simulink model "Sim"  (R2016a)
settings: Solver=VariableStepAuto  StartTime=0.0  StopTime=1500  FixedStep=1  RelTol=1e-3
values from neighbouring files (symbols this model uses):
  A = 7.841E16    (= 7.841e+16)    [Parameters.m]
  cv = 1820000    [Parameters.m]
  detaX = 0.0013333    [Parameters.m]
  Ea = 1.4766E5    (= 147660)    [Parameters.m]
  H_dr = 4.92E8    (= 492000000)    [Parameters.m]
  H_pc = 1.992E8    (= 199200000)    [Parameters.m]
  ord = 0.75    [Parameters.m]
  q_dot = 3.981E4    (= 39810)    [Parameters.m]
  T_0 = 298.15    [Parameters.m]
  Tl = 334.15    [Parameters.m]
  Ts = 331.15    [Parameters.m]
(part 1 of 3)
settings Model: Creator=pc  LastModifiedBy=pc

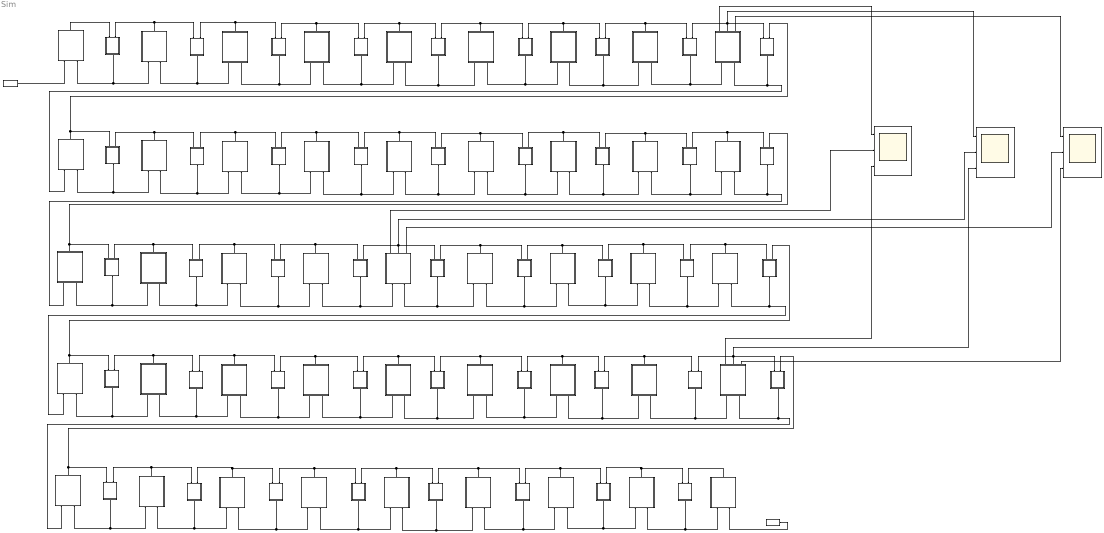
== system Sim ==
  Constant11 : Constant  Value=0
  Constant5 : Constant  Value=q_dot/detaX
  Element : Subsystem
  Element1 : Subsystem
  Element10 : Subsystem
  Element11 : Subsystem
  Element12 : Subsystem
  Element13 : Subsystem
  Element14 : Subsystem
  Element15 : Subsystem
  Element16 : Subsystem
  Element17 : Subsystem
  Element18 : Subsystem
  Element19 : Subsystem
  Element2 : Subsystem
  Element20 : Subsystem
  Element21 : Subsystem
  Element22 : Subsystem
  Element23 : Subsystem
  Element24 : Subsystem
  Element25 : Subsystem
  Element26 : Subsystem
  Element27 : Subsystem
  Element28 : Subsystem
  Element29 : Subsystem
  Element3 : Subsystem
  Element30 : Subsystem
  Element31 : Subsystem
  Element32 : Subsystem
  Element33 : Subsystem
  Element34 : Subsystem
  Element35 : Subsystem
  Element36 : Subsystem
  Element37 : Subsystem
  Element38 : Subsystem
  Element39 : Subsystem
  Element4 : Subsystem
  Element40 : Subsystem
  Element41 : Subsystem
  Element42 : Subsystem
  Element43 : Subsystem
  Element44 : Subsystem
  Element5 : Subsystem
  Element6 : Subsystem
  Element7 : Subsystem
  Element8 : Subsystem
  Element9 : Subsystem
  Heat treansfer : Subsystem
  Heat treansfer1 : Subsystem
  Heat treansfer10 : Subsystem
  Heat treansfer11 : Subsystem
  Heat treansfer12 : Subsystem
  Heat treansfer13 : Subsystem
  Heat treansfer14 : Subsystem
  Heat treansfer15 : Subsystem
  Heat treansfer16 : Subsystem
  Heat treansfer17 : Subsystem
  Heat treansfer18 : Subsystem
  Heat treansfer19 : Subsystem
  Heat treansfer2 : Subsystem
  Heat treansfer20 : Subsystem
  Heat treansfer21 : Subsystem
  Heat treansfer22 : Subsystem
  Heat treansfer23 : Subsystem
  Heat treansfer24 : Subsystem
  Heat treansfer25 : Subsystem
  Heat treansfer26 : Subsystem
  Heat treansfer27 : Subsystem
  Heat treansfer28 : Subsystem
  Heat treansfer29 : Subsystem
  Heat treansfer3 : Subsystem
  Heat treansfer30 : Subsystem
  Heat treansfer31 : Subsystem
  Heat treansfer32 : Subsystem
  Heat treansfer33 : Subsystem
  Heat treansfer34 : Subsystem
  Heat treansfer35 : Subsystem
  Heat treansfer36 : Subsystem
  Heat treansfer37 : Subsystem
  Heat treansfer38 : Subsystem
  Heat treansfer39 : Subsystem
  Heat treansfer4 : Subsystem
  Heat treansfer40 : Subsystem
  Heat treansfer41 : Subsystem
  Heat treansfer42 : Subsystem
  Heat treansfer44 : Subsystem
  Heat treansfer5 : Subsystem
  Heat treansfer6 : Subsystem
  Heat treansfer7 : Subsystem
  Heat treansfer8 : Subsystem
  Heat treansfer9 : Subsystem
  Scope : Scope  NumInputPorts=3
  Scope1 : Scope  NumInputPorts=3
  Scope2 : Scope  NumInputPorts=3
  wires:
  Constant5/1 -> Element/1(Q_in)  "Q_in"
  Element1/2(Temp) -> Heat treansfer1/1(Temp(+)), Heat treansfer/2(Temp(-))
  Heat treansfer/1(Q[W/m3]) -> Element1/1(Q_in), Element/2(Q_out)
  Heat treansfer1/1(Q[W/m3]) -> Element2/1(Q_in), Element1/2(Q_out)
  Heat treansfer2/1(Q[W/m3]) -> Element3/1(Q_in), Element2/2(Q_out)
  Heat treansfer3/1(Q[W/m3]) -> Element4/1(Q_in), Element3/2(Q_out)
  Heat treansfer4/1(Q[W/m3]) -> Element15/1(Q_in), Element4/2(Q_out)
  Element3/2(Temp) -> Heat treansfer2/2(Temp(-)), Heat treansfer3/1(Temp(+))
  Element2/2(Temp) -> Heat treansfer1/2(Temp(-)), Heat treansfer2/1(Temp(+))
  Heat treansfer14/1(Q[W/m3]) -> Element16/1(Q_in), Element15/2(Q_out)
  Heat treansfer15/1(Q[W/m3]) -> Element16/2(Q_out), Element17/1(Q_in)
  Element15/2(Temp) -> Heat treansfer14/1(Temp(+)), Heat treansfer4/2(Temp(-))
  Element16/2(Temp) -> Heat treansfer15/1(Temp(+)), Heat treansfer14/2(Temp(-))
  Element5/2(Temp) -> Heat treansfer17/2(Temp(-)), Heat treansfer5/1(Temp(+))
  Heat treansfer16/1(Q[W/m3]) -> Element18/1(Q_in), Element17/2(Q_out)
  Heat treansfer17/1(Q[W/m3]) -> Element5/1(Q_in), Element18/2(Q_out)
  Element17/2(Temp) -> Heat treansfer15/2(Temp(-)), Heat treansfer16/1(Temp(+))
  Element6/2(Temp) -> Heat treansfer6/1(Temp(+)), Heat treansfer5/2(Temp(-))
  Heat treansfer5/1(Q[W/m3]) -> Element6/1(Q_in), Element5/2(Q_out)
  Heat treansfer6/1(Q[W/m3]) -> Element20/1(Q_in), Element6/2(Q_out)
  Heat treansfer19/1(Q[W/m3]) -> Element21/1(Q_in), Element20/2(Q_out)
  Heat treansfer20/1(Q[W/m3]) -> Element22/1(Q_in), Element21/2(Q_out)
  Heat treansfer21/1(Q[W/m3]) -> Element7/1(Q_in), Element22/2(Q_out)
  Element21/2(Temp) -> Heat treansfer19/2(Temp(-)), Heat treansfer20/1(Temp(+))
  Element20/2(Temp) -> Heat treansfer6/2(Temp(-)), Heat treansfer19/1(Temp(+))
  Heat treansfer7/1(Q[W/m3]) -> Element8/1(Q_in), Element7/2(Q_out)
  Heat treansfer8/1(Q[W/m3]) -> Element8/2(Q_out), Element9/1(Q_in)
  Element7/2(Temp) -> Heat treansfer7/1(Temp(+)), Heat treansfer21/2(Temp(-))
  Element8/2(Temp) -> Heat treansfer8/1(Temp(+)), Heat treansfer7/2(Temp(-))
  Element14/2(Temp) -> Heat treansfer22/1(Temp(+)), Heat treansfer18/2(Temp(-))
  Heat treansfer9/1(Q[W/m3]) -> Element19/1(Q_in), Element9/2(Q_out)
  Heat treansfer18/1(Q[W/m3]) -> Element14/1(Q_in), Element19/2(Q_out)
  Element9/2(Temp) -> Heat treansfer8/2(Temp(-)), Heat treansfer9/1(Temp(+))
  Element19/2(Temp) -> Heat treansfer18/1(Temp(+)), Heat treansfer9/2(Temp(-))
  Element23/2(Temp) -> Heat treansfer23/1(Temp(+)), Heat treansfer22/2(Temp(-))
  Heat treansfer22/1(Q[W/m3]) -> Element23/1(Q_in), Element14/2(Q_out)
  Heat treansfer23/1(Q[W/m3]) -> Element11/1(Q_in), Element23/2(Q_out)
  Heat treansfer11/1(Q[W/m3]) -> Element12/1(Q_in), Element11/2(Q_out)
  Heat treansfer12/1(Q[W/m3]) -> Element13/1(Q_in), Element12/2(Q_out)
  Heat treansfer13/1(Q[W/m3]) -> Element24/1(Q_in), Element13/2(Q_out)
  Element12/2(Temp) -> Heat treansfer11/2(Temp(-)), Heat treansfer12/1(Temp(+))
  Element11/2(Temp) -> Heat treansfer23/2(Temp(-)), Heat treansfer11/1(Temp(+))
  Heat treansfer24/1(Q[W/m3]) -> Element25/1(Q_in), Element24/2(Q_out)
  Element24/2(Temp) -> Heat treansfer24/1(Temp(+)), Heat treansfer13/2(Temp(-))
  Element4/2(Temp) -> Heat treansfer4/1(Temp(+)), Heat treansfer3/2(Temp(-))
  Element22/2(Temp) -> Heat treansfer20/2(Temp(-)), Heat treansfer21/1(Temp(+))
  Element25/2(Temp) -> Heat treansfer26/1(Temp(+)), Heat treansfer24/2(Temp(-))
  Heat treansfer26/1(Q[W/m3]) -> Element25/2(Q_out), Element10/1(Q_in)
  Heat treansfer10/1(Q[W/m3]) -> Element26/1(Q_in), Element10/2(Q_out)
  Element26/2(Temp) -> Heat treansfer10/2(Temp(-)), Heat treansfer25/1(Temp(+))
  Element10/2(Temp) -> Heat treansfer26/2(Temp(-)), Heat treansfer10/1(Temp(+))
  Element31/2(Temp) -> Heat treansfer25/2(Temp(-)), Heat treansfer31/1(Temp(+))
  Heat treansfer25/1(Q[W/m3]) -> Element31/1(Q_in), Element26/2(Q_out)
  Element32/2(Temp) -> Heat treansfer32/1(Temp(+)), Heat treansfer31/2(Temp(-))
  Heat treansfer31/1(Q[W/m3]) -> Element32/1(Q_in), Element31/2(Q_out)
  Heat treansfer32/1(Q[W/m3]) -> Element28/1(Q_in), Element32/2(Q_out)
  Heat treansfer28/1(Q[W/m3]) -> Element29/1(Q_in), Element28/2(Q_out)
  Heat treansfer29/1(Q[W/m3]) -> Element30/1(Q_in), Element29/2(Q_out)
  Heat treansfer30/1(Q[W/m3]) -> Element33/1(Q_in), Element30/2(Q_out)
  Element29/2(Temp) -> Heat treansfer28/2(Temp(-)), Heat treansfer29/1(Temp(+))
  Element28/2(Temp) -> Heat treansfer32/2(Temp(-)), Heat treansfer28/1(Temp(+))
  Heat treansfer33/1(Q[W/m3]) -> Element34/1(Q_in), Element33/2(Q_out)
  Heat treansfer34/1(Q[W/m3]) -> Element34/2(Q_out), Element35/1(Q_in)
  Element33/2(Temp) -> Heat treansfer33/1(Temp(+)), Heat treansfer30/2(Temp(-))
  Element34/2(Temp) -> Heat treansfer34/1(Temp(+)), Heat treansfer33/2(Temp(-))
  Element35/2(Temp) -> Heat treansfer34/2(Temp(-)), Heat treansfer27/1(Temp(+))
  Element30/2(Temp) -> Heat treansfer29/2(Temp(-)), Heat treansfer30/1(Temp(+))
  Heat treansfer27/1(Q[W/m3]) -> Element35/2(Q_out), Element27/1(Q_in)
  Element40/2(Temp) -> Heat treansfer35/2(Temp(-)), Heat treansfer40/1(Temp(+))
  Heat treansfer35/1(Q[W/m3]) -> Element40/1(Q_in), Element27/2(Q_out)
  Element41/2(Temp) -> Heat treansfer41/1(Temp(+)), Heat treansfer40/2(Temp(-))
  Heat treansfer40/1(Q[W/m3]) -> Element41/1(Q_in), Element40/2(Q_out)
  Heat treansfer41/1(Q[W/m3]) -> Element37/1(Q_in), Element41/2(Q_out)
  Heat treansfer37/1(Q[W/m3]) -> Element38/1(Q_in), Element37/2(Q_out)
  Heat treansfer38/1(Q[W/m3]) -> Element39/1(Q_in), Element38/2(Q_out)
  Heat treansfer39/1(Q[W/m3]) -> Element42/1(Q_in), Element39/2(Q_out)
  Element38/2(Temp) -> Heat treansfer37/2(Temp(-)), Heat treansfer38/1(Temp(+))
  Element37/2(Temp) -> Heat treansfer41/2(Temp(-)), Heat treansfer37/1(Temp(+))
  Heat treansfer42/1(Q[W/m3]) -> Element43/1(Q_in), Element42/2(Q_out)
  Element42/2(Temp) -> Heat treansfer42/1(Temp(+)), Heat treansfer39/2(Temp(-))
  Element39/2(Temp) -> Heat treansfer38/2(Temp(-)), Heat treansfer39/1(Temp(+))
  Element43/2(Temp) -> Heat treansfer44/1(Temp(+)), Heat treansfer42/2(Temp(-))
  Heat treansfer44/1(Q[W/m3]) -> Element43/2(Q_out), Element36/1(Q_in)
  Heat treansfer36/1(Q[W/m3]) -> Element44/1(Q_in), Element36/2(Q_out)
  Element36/2(Temp) -> Heat treansfer44/2(Temp(-)), Heat treansfer36/1(Temp(+))
  Constant11/1 -> Element44/2(Q_out)
  Element13/1(Beta) -> Scope/2
  Element13/3(Alpha) -> Scope2/2
  Element13/2(Temp) -> Scope1/2, Heat treansfer12/2(Temp(-)), Heat treansfer13/1(Temp(+))
  Element/2(Temp) -> Heat treansfer/1(Temp(+))
  Element44/2(Temp) -> Heat treansfer36/2(Temp(-))
  Element18/1(Beta) -> Scope/1
  Element18/2(Temp) -> Scope1/1, Heat treansfer17/1(Temp(+)), Heat treansfer16/2(Temp(-))
  Element18/3(Alpha) -> Scope2/1
  Element27/1(Beta) -> Scope/3
  Element27/2(Temp) -> Scope1/3, Heat treansfer35/1(Temp(+)), Heat treansfer27/2(Temp(-))
  Element27/3(Alpha) -> Scope2/3

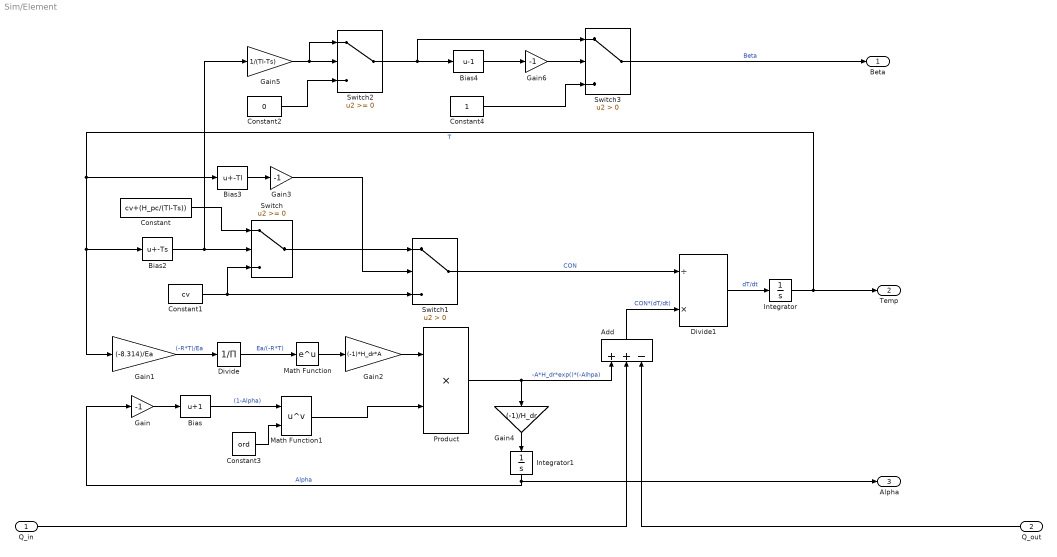
== system Sim/Element ==
  Q_in : Inport
  Q_out : Inport  Port=2
  Add : Sum  Inputs=++-
  Bias : Bias  Bias=1
  Bias2 : Bias  Bias=-Ts
  Bias3 : Bias  Bias=-Tl
  Bias4 : Bias  Bias=-1
  Constant : Constant  Value=cv+(H_pc/(Tl-Ts))
  Constant1 : Constant  Value=cv
  Constant2 : Constant  Value=0
  Constant3 : Constant  Value=ord
  Constant4 : Constant
  Divide : Product  Inputs=/
  Divide1 : Product  Inputs=/*
  Gain : Gain  Gain=-1
  Gain1 : Gain  Gain=(-8.314)/Ea
  Gain2 : Gain  Gain=(-1)*H_dr*A
  Gain3 : Gain  Gain=-1
  Gain4 : Gain  Gain=(-1)/H_dr
  Gain5 : Gain  Gain=1/(Tl-Ts)
  Gain6 : Gain  Gain=-1
  Integrator : Integrator  InitialCondition=T_0
  Integrator1 : Integrator
  Math Function : Math  SaturateOnIntegerOverflow=on
  Math Function1 : Math  Operator=pow  SaturateOnIntegerOverflow=on
  Product : Product
  Switch : Switch
  Switch1 : Switch  Criteria=u2 > Threshold
  Switch2 : Switch
  Switch3 : Switch  Criteria=u2 > Threshold
  Beta : Outport
  Temp : Outport  Port=2
  Alpha : Outport  Port=3
  wires:
  Q_out/1 -> Add/3
  Gain/1 -> Bias/1
  Divide1/1 -> Integrator/1  "dT/dt"
  Gain2/1 -> Product/1
  Integrator/1 -> Temp/1, Bias3/1, Bias2/1, Gain1/1  "T"
  Switch1/1 -> Divide1/1  "CON"
  Math Function1/1 -> Product/2
  Bias/1 -> Math Function1/1  "(1-Alpha)"
  Constant2/1 -> Switch2/3
  Add/1 -> Divide1/2  "CON*(dT/dt)"
  Gain5/1 -> Switch2/1, Switch2/2
  Switch2/1 -> Switch3/1, Bias4/1
  Constant/1 -> Switch/1
  Bias4/1 -> Gain6/1
  Switch/1 -> Switch1/1
  Switch3/1 -> Beta/1  "Beta"
  Gain6/1 -> Switch3/2
  Bias2/1 -> Gain5/1, Switch/2
  Constant4/1 -> Switch3/3
  Product/1 -> Add/1, Gain4/1  "-A*H_dr*exp()*(-Alhpa)"
  Gain1/1 -> Divide/1  "(-R*T)/Ea"
  Integrator1/1 -> Gain/1, Alpha/1  "Alpha"
  Gain4/1 -> Integrator1/1
  Constant3/1 -> Math Function1/2
  Constant1/1 -> Switch/3, Switch1/3
  Divide/1 -> Math Function/1  "Ea/(-R*T)"
  Math Function/1 -> Gain2/1
  Bias3/1 -> Gain3/1
  Gain3/1 -> Switch1/2
  Q_in/1 -> Add/2

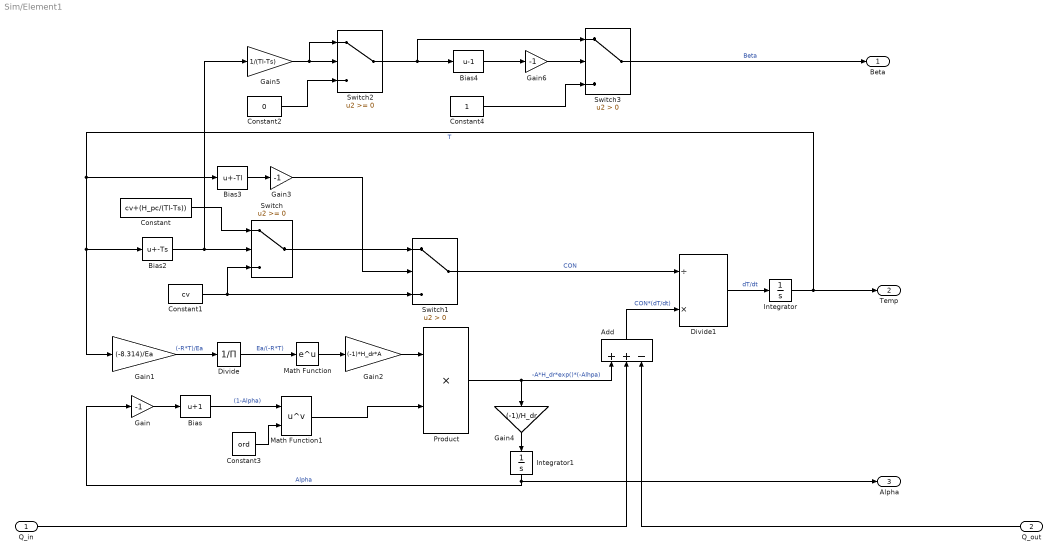
== system Sim/Element1 ==
  Q_in : Inport
  Q_out : Inport  Port=2
  Add : Sum  Inputs=++-
  Bias : Bias  Bias=1
  Bias2 : Bias  Bias=-Ts
  Bias3 : Bias  Bias=-Tl
  Bias4 : Bias  Bias=-1
  Constant : Constant  Value=cv+(H_pc/(Tl-Ts))
  Constant1 : Constant  Value=cv
  Constant2 : Constant  Value=0
  Constant3 : Constant  Value=ord
  Constant4 : Constant
  Divide : Product  Inputs=/
  Divide1 : Product  Inputs=/*
  Gain : Gain  Gain=-1
  Gain1 : Gain  Gain=(-8.314)/Ea
  Gain2 : Gain  Gain=(-1)*H_dr*A
  Gain3 : Gain  Gain=-1
  Gain4 : Gain  Gain=(-1)/H_dr
  Gain5 : Gain  Gain=1/(Tl-Ts)
  Gain6 : Gain  Gain=-1
  Integrator : Integrator  InitialCondition=T_0
  Integrator1 : Integrator
  Math Function : Math  SaturateOnIntegerOverflow=on
  Math Function1 : Math  Operator=pow  SaturateOnIntegerOverflow=on
  Product : Product
  Switch : Switch
  Switch1 : Switch  Criteria=u2 > Threshold
  Switch2 : Switch
  Switch3 : Switch  Criteria=u2 > Threshold
  Beta : Outport
  Temp : Outport  Port=2
  Alpha : Outport  Port=3
  wires:
  Q_out/1 -> Add/3
  Gain/1 -> Bias/1
  Divide1/1 -> Integrator/1  "dT/dt"
  Gain2/1 -> Product/1
  Integrator/1 -> Temp/1, Bias3/1, Bias2/1, Gain1/1  "T"
  Switch1/1 -> Divide1/1  "CON"
  Math Function1/1 -> Product/2
  Bias/1 -> Math Function1/1  "(1-Alpha)"
  Constant2/1 -> Switch2/3
  Add/1 -> Divide1/2  "CON*(dT/dt)"
  Gain5/1 -> Switch2/1, Switch2/2
  Switch2/1 -> Switch3/1, Bias4/1
  Constant/1 -> Switch/1
  Bias4/1 -> Gain6/1
  Switch/1 -> Switch1/1
  Switch3/1 -> Beta/1  "Beta"
  Gain6/1 -> Switch3/2
  Bias2/1 -> Gain5/1, Switch/2
  Constant4/1 -> Switch3/3
  Product/1 -> Add/1, Gain4/1  "-A*H_dr*exp()*(-Alhpa)"
  Gain1/1 -> Divide/1  "(-R*T)/Ea"
  Integrator1/1 -> Gain/1, Alpha/1  "Alpha"
  Gain4/1 -> Integrator1/1
  Constant3/1 -> Math Function1/2
  Constant1/1 -> Switch/3, Switch1/3
  Divide/1 -> Math Function/1  "Ea/(-R*T)"
  Math Function/1 -> Gain2/1
  Bias3/1 -> Gain3/1
  Gain3/1 -> Switch1/2
  Q_in/1 -> Add/2

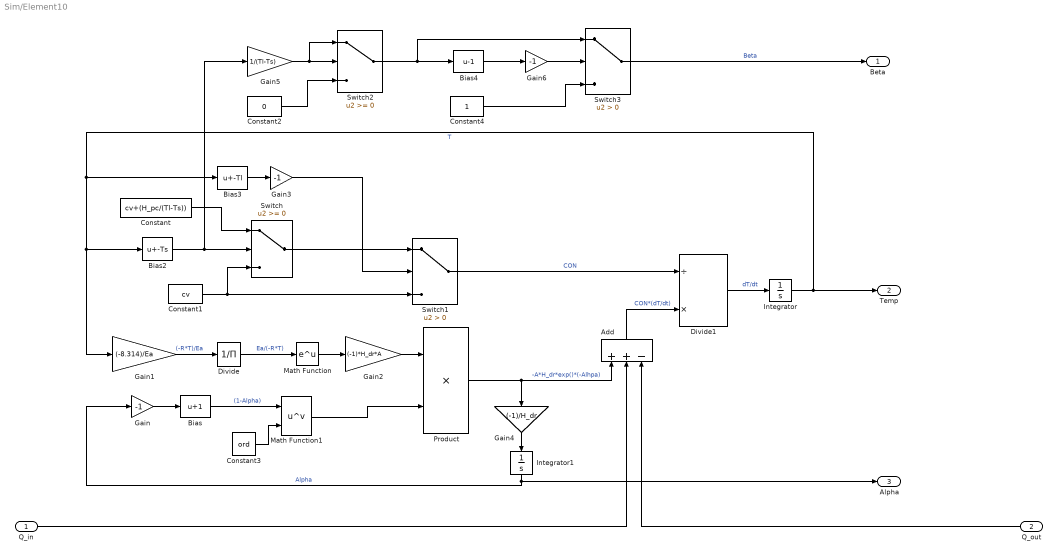
== system Sim/Element10 ==
  Q_in : Inport
  Q_out : Inport  Port=2
  Add : Sum  Inputs=++-
  Bias : Bias  Bias=1
  Bias2 : Bias  Bias=-Ts
  Bias3 : Bias  Bias=-Tl
  Bias4 : Bias  Bias=-1
  Constant : Constant  Value=cv+(H_pc/(Tl-Ts))
  Constant1 : Constant  Value=cv
  Constant2 : Constant  Value=0
  Constant3 : Constant  Value=ord
  Constant4 : Constant
  Divide : Product  Inputs=/
  Divide1 : Product  Inputs=/*
  Gain : Gain  Gain=-1
  Gain1 : Gain  Gain=(-8.314)/Ea
  Gain2 : Gain  Gain=(-1)*H_dr*A
  Gain3 : Gain  Gain=-1
  Gain4 : Gain  Gain=(-1)/H_dr
  Gain5 : Gain  Gain=1/(Tl-Ts)
  Gain6 : Gain  Gain=-1
  Integrator : Integrator  InitialCondition=T_0
  Integrator1 : Integrator
  Math Function : Math  SaturateOnIntegerOverflow=on
  Math Function1 : Math  Operator=pow  SaturateOnIntegerOverflow=on
  Product : Product
  Switch : Switch
  Switch1 : Switch  Criteria=u2 > Threshold
  Switch2 : Switch
  Switch3 : Switch  Criteria=u2 > Threshold
  Beta : Outport
  Temp : Outport  Port=2
  Alpha : Outport  Port=3
  wires:
  Q_out/1 -> Add/3
  Gain/1 -> Bias/1
  Divide1/1 -> Integrator/1  "dT/dt"
  Gain2/1 -> Product/1
  Integrator/1 -> Temp/1, Bias3/1, Bias2/1, Gain1/1  "T"
  Switch1/1 -> Divide1/1  "CON"
  Math Function1/1 -> Product/2
  Bias/1 -> Math Function1/1  "(1-Alpha)"
  Constant2/1 -> Switch2/3
  Add/1 -> Divide1/2  "CON*(dT/dt)"
  Gain5/1 -> Switch2/1, Switch2/2
  Switch2/1 -> Switch3/1, Bias4/1
  Constant/1 -> Switch/1
  Bias4/1 -> Gain6/1
  Switch/1 -> Switch1/1
  Switch3/1 -> Beta/1  "Beta"
  Gain6/1 -> Switch3/2
  Bias2/1 -> Gain5/1, Switch/2
  Constant4/1 -> Switch3/3
  Product/1 -> Add/1, Gain4/1  "-A*H_dr*exp()*(-Alhpa)"
  Gain1/1 -> Divide/1  "(-R*T)/Ea"
  Integrator1/1 -> Gain/1, Alpha/1  "Alpha"
  Gain4/1 -> Integrator1/1
  Constant3/1 -> Math Function1/2
  Constant1/1 -> Switch/3, Switch1/3
  Divide/1 -> Math Function/1  "Ea/(-R*T)"
  Math Function/1 -> Gain2/1
  Bias3/1 -> Gain3/1
  Gain3/1 -> Switch1/2
  Q_in/1 -> Add/2

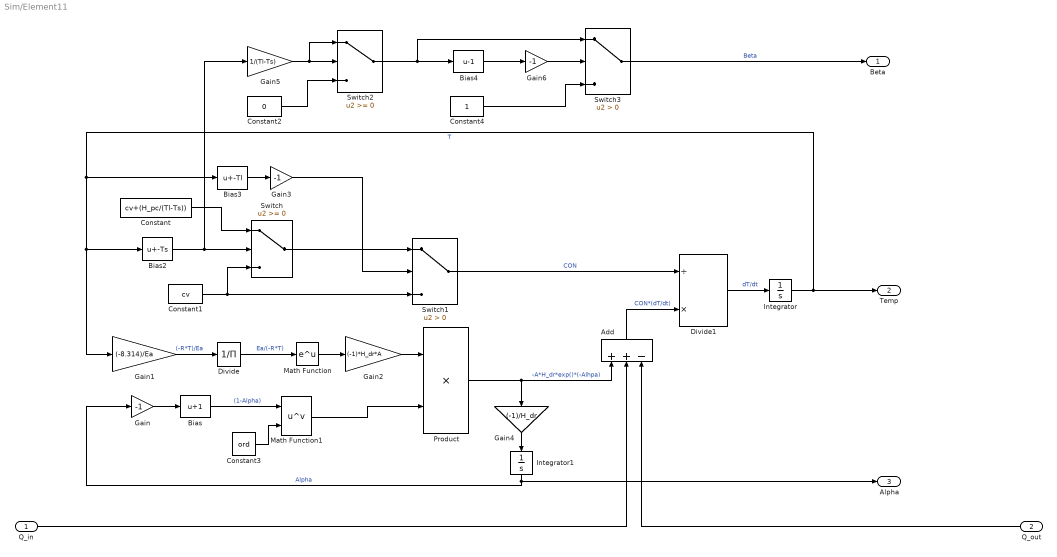
== system Sim/Element11 ==
  Q_in : Inport
  Q_out : Inport  Port=2
  Add : Sum  Inputs=++-
  Bias : Bias  Bias=1
  Bias2 : Bias  Bias=-Ts
  Bias3 : Bias  Bias=-Tl
  Bias4 : Bias  Bias=-1
  Constant : Constant  Value=cv+(H_pc/(Tl-Ts))
  Constant1 : Constant  Value=cv
  Constant2 : Constant  Value=0
  Constant3 : Constant  Value=ord
  Constant4 : Constant
  Divide : Product  Inputs=/
  Divide1 : Product  Inputs=/*
  Gain : Gain  Gain=-1
  Gain1 : Gain  Gain=(-8.314)/Ea
  Gain2 : Gain  Gain=(-1)*H_dr*A
  Gain3 : Gain  Gain=-1
  Gain4 : Gain  Gain=(-1)/H_dr
  Gain5 : Gain  Gain=1/(Tl-Ts)
  Gain6 : Gain  Gain=-1
  Integrator : Integrator  InitialCondition=T_0
  Integrator1 : Integrator
  Math Function : Math  SaturateOnIntegerOverflow=on
  Math Function1 : Math  Operator=pow  SaturateOnIntegerOverflow=on
  Product : Product
  Switch : Switch
  Switch1 : Switch  Criteria=u2 > Threshold
  Switch2 : Switch
  Switch3 : Switch  Criteria=u2 > Threshold
  Beta : Outport
  Temp : Outport  Port=2
  Alpha : Outport  Port=3
  wires:
  Q_out/1 -> Add/3
  Gain/1 -> Bias/1
  Divide1/1 -> Integrator/1  "dT/dt"
  Gain2/1 -> Product/1
  Integrator/1 -> Temp/1, Bias3/1, Bias2/1, Gain1/1  "T"
  Switch1/1 -> Divide1/1  "CON"
  Math Function1/1 -> Product/2
  Bias/1 -> Math Function1/1  "(1-Alpha)"
  Constant2/1 -> Switch2/3
  Add/1 -> Divide1/2  "CON*(dT/dt)"
  Gain5/1 -> Switch2/1, Switch2/2
  Switch2/1 -> Switch3/1, Bias4/1
  Constant/1 -> Switch/1
  Bias4/1 -> Gain6/1
  Switch/1 -> Switch1/1
  Switch3/1 -> Beta/1  "Beta"
  Gain6/1 -> Switch3/2
  Bias2/1 -> Gain5/1, Switch/2
  Constant4/1 -> Switch3/3
  Product/1 -> Add/1, Gain4/1  "-A*H_dr*exp()*(-Alhpa)"
  Gain1/1 -> Divide/1  "(-R*T)/Ea"
  Integrator1/1 -> Gain/1, Alpha/1  "Alpha"
  Gain4/1 -> Integrator1/1
  Constant3/1 -> Math Function1/2
  Constant1/1 -> Switch/3, Switch1/3
  Divide/1 -> Math Function/1  "Ea/(-R*T)"
  Math Function/1 -> Gain2/1
  Bias3/1 -> Gain3/1
  Gain3/1 -> Switch1/2
  Q_in/1 -> Add/2

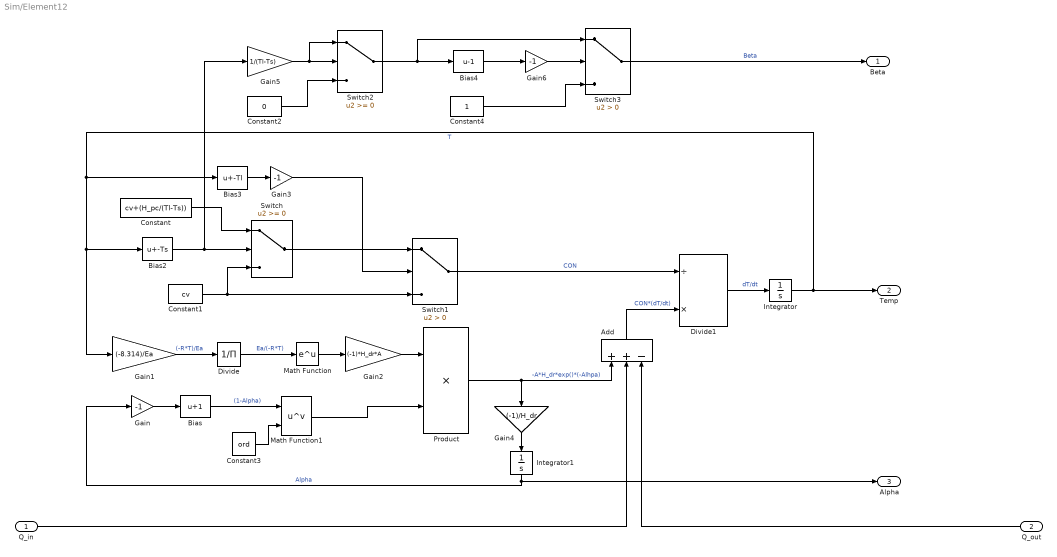
== system Sim/Element12 ==
  Q_in : Inport
  Q_out : Inport  Port=2
  Add : Sum  Inputs=++-
  Bias : Bias  Bias=1
  Bias2 : Bias  Bias=-Ts
  Bias3 : Bias  Bias=-Tl
  Bias4 : Bias  Bias=-1
  Constant : Constant  Value=cv+(H_pc/(Tl-Ts))
  Constant1 : Constant  Value=cv
  Constant2 : Constant  Value=0
  Constant3 : Constant  Value=ord
  Constant4 : Constant
  Divide : Product  Inputs=/
  Divide1 : Product  Inputs=/*
  Gain : Gain  Gain=-1
  Gain1 : Gain  Gain=(-8.314)/Ea
  Gain2 : Gain  Gain=(-1)*H_dr*A
  Gain3 : Gain  Gain=-1
  Gain4 : Gain  Gain=(-1)/H_dr
  Gain5 : Gain  Gain=1/(Tl-Ts)
  Gain6 : Gain  Gain=-1
  Integrator : Integrator  InitialCondition=T_0
  Integrator1 : Integrator
  Math Function : Math  SaturateOnIntegerOverflow=on
  Math Function1 : Math  Operator=pow  SaturateOnIntegerOverflow=on
  Product : Product
  Switch : Switch
  Switch1 : Switch  Criteria=u2 > Threshold
  Switch2 : Switch
  Switch3 : Switch  Criteria=u2 > Threshold
  Beta : Outport
  Temp : Outport  Port=2
  Alpha : Outport  Port=3
  wires:
  Q_out/1 -> Add/3
  Gain/1 -> Bias/1
  Divide1/1 -> Integrator/1  "dT/dt"
  Gain2/1 -> Product/1
  Integrator/1 -> Temp/1, Bias3/1, Bias2/1, Gain1/1  "T"
  Switch1/1 -> Divide1/1  "CON"
  Math Function1/1 -> Product/2
  Bias/1 -> Math Function1/1  "(1-Alpha)"
  Constant2/1 -> Switch2/3
  Add/1 -> Divide1/2  "CON*(dT/dt)"
  Gain5/1 -> Switch2/1, Switch2/2
  Switch2/1 -> Switch3/1, Bias4/1
  Constant/1 -> Switch/1
  Bias4/1 -> Gain6/1
  Switch/1 -> Switch1/1
  Switch3/1 -> Beta/1  "Beta"
  Gain6/1 -> Switch3/2
  Bias2/1 -> Gain5/1, Switch/2
  Constant4/1 -> Switch3/3
  Product/1 -> Add/1, Gain4/1  "-A*H_dr*exp()*(-Alhpa)"
  Gain1/1 -> Divide/1  "(-R*T)/Ea"
  Integrator1/1 -> Gain/1, Alpha/1  "Alpha"
  Gain4/1 -> Integrator1/1
  Constant3/1 -> Math Function1/2
  Constant1/1 -> Switch/3, Switch1/3
  Divide/1 -> Math Function/1  "Ea/(-R*T)"
  Math Function/1 -> Gain2/1
  Bias3/1 -> Gain3/1
  Gain3/1 -> Switch1/2
  Q_in/1 -> Add/2

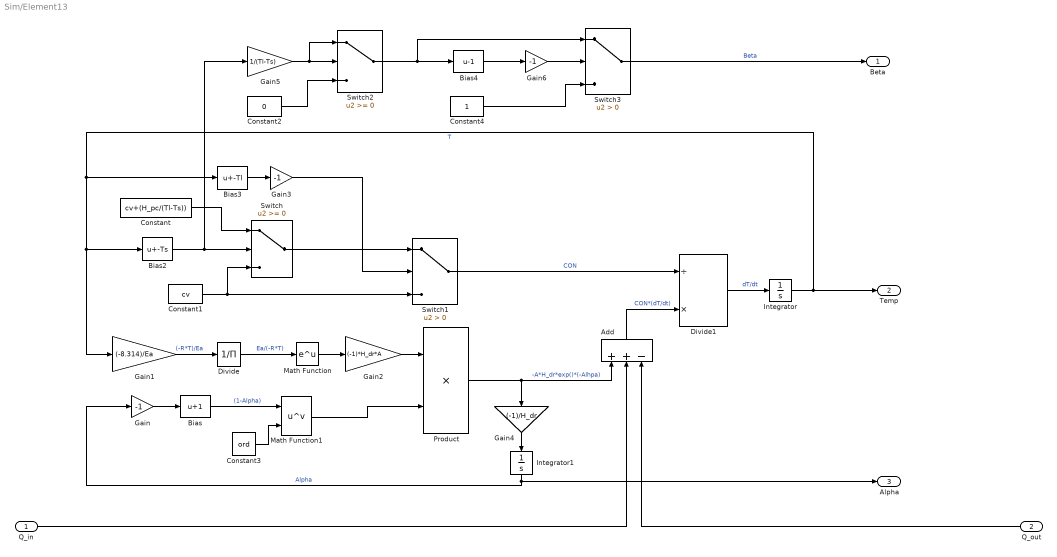
== system Sim/Element13 ==
  Q_in : Inport
  Q_out : Inport  Port=2
  Add : Sum  Inputs=++-
  Bias : Bias  Bias=1
  Bias2 : Bias  Bias=-Ts
  Bias3 : Bias  Bias=-Tl
  Bias4 : Bias  Bias=-1
  Constant : Constant  Value=cv+(H_pc/(Tl-Ts))
  Constant1 : Constant  Value=cv
  Constant2 : Constant  Value=0
  Constant3 : Constant  Value=ord
  Constant4 : Constant
  Divide : Product  Inputs=/
  Divide1 : Product  Inputs=/*
  Gain : Gain  Gain=-1
  Gain1 : Gain  Gain=(-8.314)/Ea
  Gain2 : Gain  Gain=(-1)*H_dr*A
  Gain3 : Gain  Gain=-1
  Gain4 : Gain  Gain=(-1)/H_dr
  Gain5 : Gain  Gain=1/(Tl-Ts)
  Gain6 : Gain  Gain=-1
  Integrator : Integrator  InitialCondition=T_0
  Integrator1 : Integrator
  Math Function : Math  SaturateOnIntegerOverflow=on
  Math Function1 : Math  Operator=pow  SaturateOnIntegerOverflow=on
  Product : Product
  Switch : Switch
  Switch1 : Switch  Criteria=u2 > Threshold
  Switch2 : Switch
  Switch3 : Switch  Criteria=u2 > Threshold
  Beta : Outport
  Temp : Outport  Port=2
  Alpha : Outport  Port=3
  wires:
  Q_out/1 -> Add/3
  Gain/1 -> Bias/1
  Divide1/1 -> Integrator/1  "dT/dt"
  Gain2/1 -> Product/1
  Integrator/1 -> Temp/1, Bias3/1, Bias2/1, Gain1/1  "T"
  Switch1/1 -> Divide1/1  "CON"
  Math Function1/1 -> Product/2
  Bias/1 -> Math Function1/1  "(1-Alpha)"
  Constant2/1 -> Switch2/3
  Add/1 -> Divide1/2  "CON*(dT/dt)"
  Gain5/1 -> Switch2/1, Switch2/2
  Switch2/1 -> Switch3/1, Bias4/1
  Constant/1 -> Switch/1
  Bias4/1 -> Gain6/1
  Switch/1 -> Switch1/1
  Switch3/1 -> Beta/1  "Beta"
  Gain6/1 -> Switch3/2
  Bias2/1 -> Gain5/1, Switch/2
  Constant4/1 -> Switch3/3
  Product/1 -> Add/1, Gain4/1  "-A*H_dr*exp()*(-Alhpa)"
  Gain1/1 -> Divide/1  "(-R*T)/Ea"
  Integrator1/1 -> Gain/1, Alpha/1  "Alpha"
  Gain4/1 -> Integrator1/1
  Constant3/1 -> Math Function1/2
  Constant1/1 -> Switch/3, Switch1/3
  Divide/1 -> Math Function/1  "Ea/(-R*T)"
  Math Function/1 -> Gain2/1
  Bias3/1 -> Gain3/1
  Gain3/1 -> Switch1/2
  Q_in/1 -> Add/2

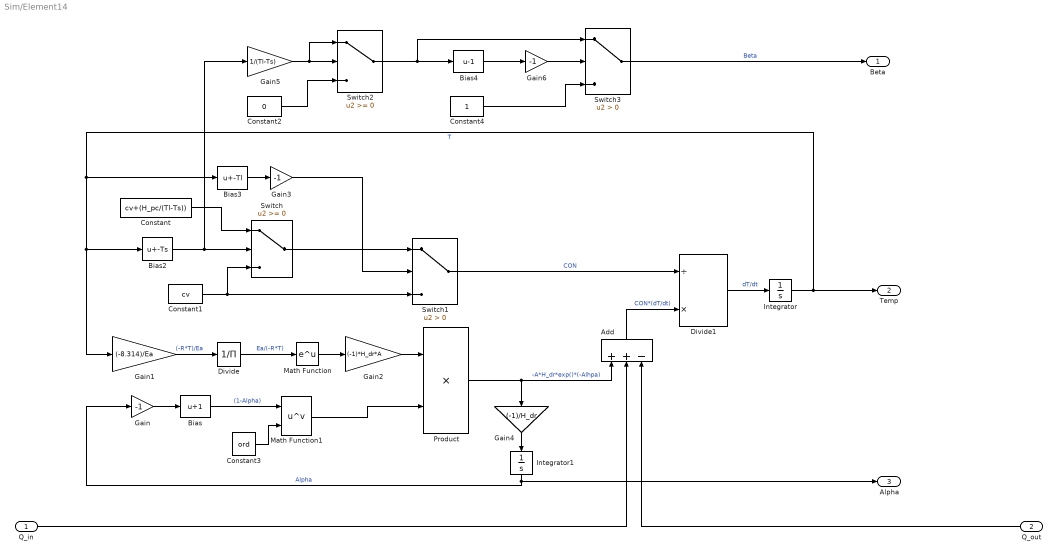
== system Sim/Element14 ==
  Q_in : Inport
  Q_out : Inport  Port=2
  Add : Sum  Inputs=++-
  Bias : Bias  Bias=1
  Bias2 : Bias  Bias=-Ts
  Bias3 : Bias  Bias=-Tl
  Bias4 : Bias  Bias=-1
  Constant : Constant  Value=cv+(H_pc/(Tl-Ts))
  Constant1 : Constant  Value=cv
  Constant2 : Constant  Value=0
  Constant3 : Constant  Value=ord
  Constant4 : Constant
  Divide : Product  Inputs=/
  Divide1 : Product  Inputs=/*
  Gain : Gain  Gain=-1
  Gain1 : Gain  Gain=(-8.314)/Ea
  Gain2 : Gain  Gain=(-1)*H_dr*A
  Gain3 : Gain  Gain=-1
  Gain4 : Gain  Gain=(-1)/H_dr
  Gain5 : Gain  Gain=1/(Tl-Ts)
  Gain6 : Gain  Gain=-1
  Integrator : Integrator  InitialCondition=T_0
  Integrator1 : Integrator
  Math Function : Math  SaturateOnIntegerOverflow=on
  Math Function1 : Math  Operator=pow  SaturateOnIntegerOverflow=on
  Product : Product
  Switch : Switch
  Switch1 : Switch  Criteria=u2 > Threshold
  Switch2 : Switch
  Switch3 : Switch  Criteria=u2 > Threshold
  Beta : Outport
  Temp : Outport  Port=2
  Alpha : Outport  Port=3
  wires:
  Q_out/1 -> Add/3
  Gain/1 -> Bias/1
  Divide1/1 -> Integrator/1  "dT/dt"
  Gain2/1 -> Product/1
  Integrator/1 -> Temp/1, Bias3/1, Bias2/1, Gain1/1  "T"
  Switch1/1 -> Divide1/1  "CON"
  Math Function1/1 -> Product/2
  Bias/1 -> Math Function1/1  "(1-Alpha)"
  Constant2/1 -> Switch2/3
  Add/1 -> Divide1/2  "CON*(dT/dt)"
  Gain5/1 -> Switch2/1, Switch2/2
  Switch2/1 -> Switch3/1, Bias4/1
  Constant/1 -> Switch/1
  Bias4/1 -> Gain6/1
  Switch/1 -> Switch1/1
  Switch3/1 -> Beta/1  "Beta"
  Gain6/1 -> Switch3/2
  Bias2/1 -> Gain5/1, Switch/2
  Constant4/1 -> Switch3/3
  Product/1 -> Add/1, Gain4/1  "-A*H_dr*exp()*(-Alhpa)"
  Gain1/1 -> Divide/1  "(-R*T)/Ea"
  Integrator1/1 -> Gain/1, Alpha/1  "Alpha"
  Gain4/1 -> Integrator1/1
  Constant3/1 -> Math Function1/2
  Constant1/1 -> Switch/3, Switch1/3
  Divide/1 -> Math Function/1  "Ea/(-R*T)"
  Math Function/1 -> Gain2/1
  Bias3/1 -> Gain3/1
  Gain3/1 -> Switch1/2
  Q_in/1 -> Add/2

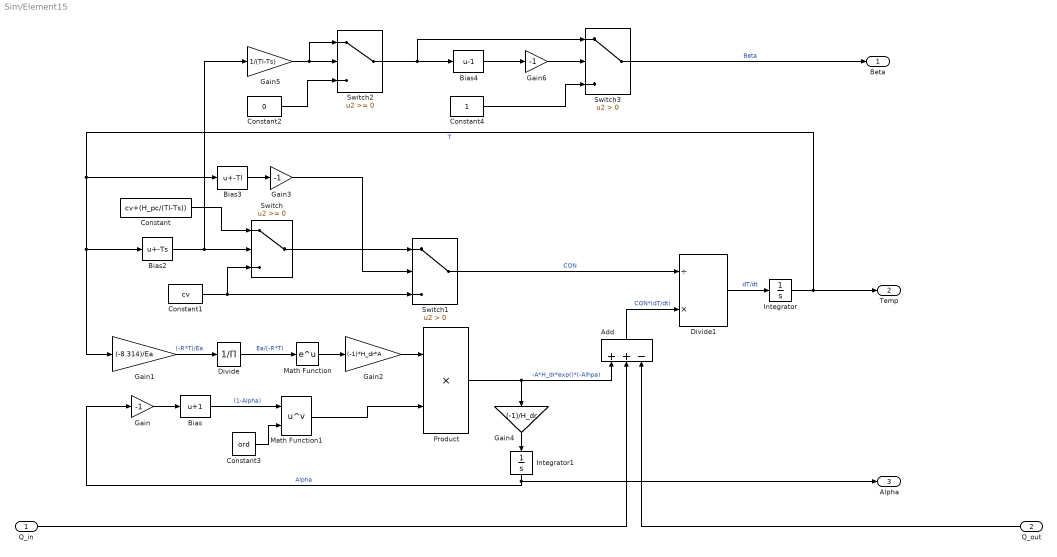
== system Sim/Element15 ==
  Q_in : Inport
  Q_out : Inport  Port=2
  Add : Sum  Inputs=++-
  Bias : Bias  Bias=1
  Bias2 : Bias  Bias=-Ts
  Bias3 : Bias  Bias=-Tl
  Bias4 : Bias  Bias=-1
  Constant : Constant  Value=cv+(H_pc/(Tl-Ts))
  Constant1 : Constant  Value=cv
  Constant2 : Constant  Value=0
  Constant3 : Constant  Value=ord
  Constant4 : Constant
  Divide : Product  Inputs=/
  Divide1 : Product  Inputs=/*
  Gain : Gain  Gain=-1
  Gain1 : Gain  Gain=(-8.314)/Ea
  Gain2 : Gain  Gain=(-1)*H_dr*A
  Gain3 : Gain  Gain=-1
  Gain4 : Gain  Gain=(-1)/H_dr
  Gain5 : Gain  Gain=1/(Tl-Ts)
  Gain6 : Gain  Gain=-1
  Integrator : Integrator  InitialCondition=T_0
  Integrator1 : Integrator
  Math Function : Math  SaturateOnIntegerOverflow=on
  Math Function1 : Math  Operator=pow  SaturateOnIntegerOverflow=on
  Product : Product
  Switch : Switch
  Switch1 : Switch  Criteria=u2 > Threshold
  Switch2 : Switch
  Switch3 : Switch  Criteria=u2 > Threshold
  Beta : Outport
  Temp : Outport  Port=2
  Alpha : Outport  Port=3
  wires:
  Q_out/1 -> Add/3
  Gain/1 -> Bias/1
  Divide1/1 -> Integrator/1  "dT/dt"
  Gain2/1 -> Product/1
  Integrator/1 -> Temp/1, Bias3/1, Bias2/1, Gain1/1  "T"
  Switch1/1 -> Divide1/1  "CON"
  Math Function1/1 -> Product/2
  Bias/1 -> Math Function1/1  "(1-Alpha)"
  Constant2/1 -> Switch2/3
  Add/1 -> Divide1/2  "CON*(dT/dt)"
  Gain5/1 -> Switch2/1, Switch2/2
  Switch2/1 -> Switch3/1, Bias4/1
  Constant/1 -> Switch/1
  Bias4/1 -> Gain6/1
  Switch/1 -> Switch1/1
  Switch3/1 -> Beta/1  "Beta"
  Gain6/1 -> Switch3/2
  Bias2/1 -> Gain5/1, Switch/2
  Constant4/1 -> Switch3/3
  Product/1 -> Add/1, Gain4/1  "-A*H_dr*exp()*(-Alhpa)"
  Gain1/1 -> Divide/1  "(-R*T)/Ea"
  Integrator1/1 -> Gain/1, Alpha/1  "Alpha"
  Gain4/1 -> Integrator1/1
  Constant3/1 -> Math Function1/2
  Constant1/1 -> Switch/3, Switch1/3
  Divide/1 -> Math Function/1  "Ea/(-R*T)"
  Math Function/1 -> Gain2/1
  Bias3/1 -> Gain3/1
  Gain3/1 -> Switch1/2
  Q_in/1 -> Add/2

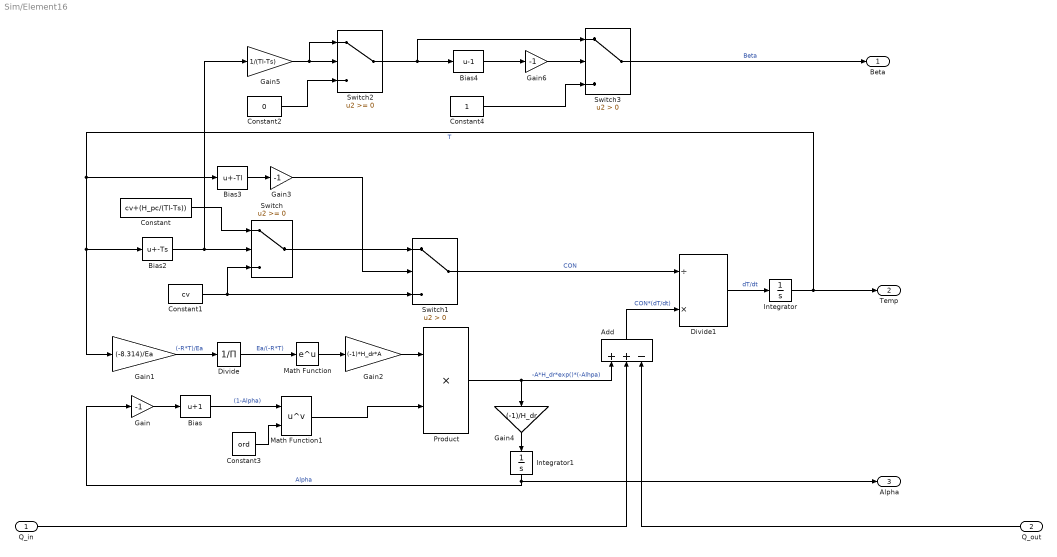
== system Sim/Element16 ==
  Q_in : Inport
  Q_out : Inport  Port=2
  Add : Sum  Inputs=++-
  Bias : Bias  Bias=1
  Bias2 : Bias  Bias=-Ts
  Bias3 : Bias  Bias=-Tl
  Bias4 : Bias  Bias=-1
  Constant : Constant  Value=cv+(H_pc/(Tl-Ts))
  Constant1 : Constant  Value=cv
  Constant2 : Constant  Value=0
  Constant3 : Constant  Value=ord
  Constant4 : Constant
  Divide : Product  Inputs=/
  Divide1 : Product  Inputs=/*
  Gain : Gain  Gain=-1
  Gain1 : Gain  Gain=(-8.314)/Ea
  Gain2 : Gain  Gain=(-1)*H_dr*A
  Gain3 : Gain  Gain=-1
  Gain4 : Gain  Gain=(-1)/H_dr
  Gain5 : Gain  Gain=1/(Tl-Ts)
  Gain6 : Gain  Gain=-1
  Integrator : Integrator  InitialCondition=T_0
  Integrator1 : Integrator
  Math Function : Math  SaturateOnIntegerOverflow=on
  Math Function1 : Math  Operator=pow  SaturateOnIntegerOverflow=on
  Product : Product
  Switch : Switch
  Switch1 : Switch  Criteria=u2 > Threshold
  Switch2 : Switch
  Switch3 : Switch  Criteria=u2 > Threshold
  Beta : Outport
  Temp : Outport  Port=2
  Alpha : Outport  Port=3
  wires:
  Q_out/1 -> Add/3
  Gain/1 -> Bias/1
  Divide1/1 -> Integrator/1  "dT/dt"
  Gain2/1 -> Product/1
  Integrator/1 -> Temp/1, Bias3/1, Bias2/1, Gain1/1  "T"
  Switch1/1 -> Divide1/1  "CON"
  Math Function1/1 -> Product/2
  Bias/1 -> Math Function1/1  "(1-Alpha)"
  Constant2/1 -> Switch2/3
  Add/1 -> Divide1/2  "CON*(dT/dt)"
  Gain5/1 -> Switch2/1, Switch2/2
  Switch2/1 -> Switch3/1, Bias4/1
  Constant/1 -> Switch/1
  Bias4/1 -> Gain6/1
  Switch/1 -> Switch1/1
  Switch3/1 -> Beta/1  "Beta"
  Gain6/1 -> Switch3/2
  Bias2/1 -> Gain5/1, Switch/2
  Constant4/1 -> Switch3/3
  Product/1 -> Add/1, Gain4/1  "-A*H_dr*exp()*(-Alhpa)"
  Gain1/1 -> Divide/1  "(-R*T)/Ea"
  Integrator1/1 -> Gain/1, Alpha/1  "Alpha"
  Gain4/1 -> Integrator1/1
  Constant3/1 -> Math Function1/2
  Constant1/1 -> Switch/3, Switch1/3
  Divide/1 -> Math Function/1  "Ea/(-R*T)"
  Math Function/1 -> Gain2/1
  Bias3/1 -> Gain3/1
  Gain3/1 -> Switch1/2
  Q_in/1 -> Add/2

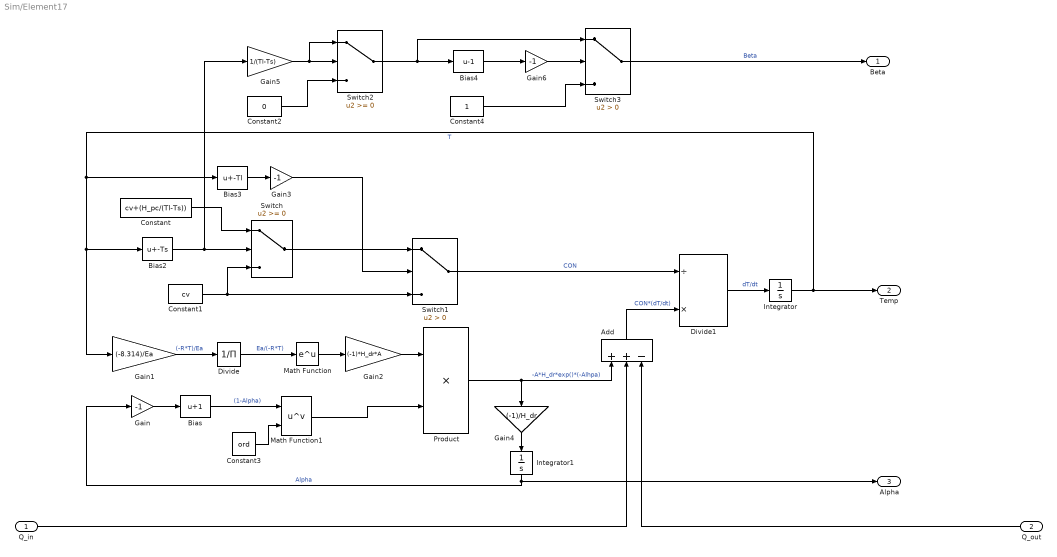
== system Sim/Element17 ==
  Q_in : Inport
  Q_out : Inport  Port=2
  Add : Sum  Inputs=++-
  Bias : Bias  Bias=1
  Bias2 : Bias  Bias=-Ts
  Bias3 : Bias  Bias=-Tl
  Bias4 : Bias  Bias=-1
  Constant : Constant  Value=cv+(H_pc/(Tl-Ts))
  Constant1 : Constant  Value=cv
  Constant2 : Constant  Value=0
  Constant3 : Constant  Value=ord
  Constant4 : Constant
  Divide : Product  Inputs=/
  Divide1 : Product  Inputs=/*
  Gain : Gain  Gain=-1
  Gain1 : Gain  Gain=(-8.314)/Ea
  Gain2 : Gain  Gain=(-1)*H_dr*A
  Gain3 : Gain  Gain=-1
  Gain4 : Gain  Gain=(-1)/H_dr
  Gain5 : Gain  Gain=1/(Tl-Ts)
  Gain6 : Gain  Gain=-1
  Integrator : Integrator  InitialCondition=T_0
  Integrator1 : Integrator
  Math Function : Math  SaturateOnIntegerOverflow=on
  Math Function1 : Math  Operator=pow  SaturateOnIntegerOverflow=on
  Product : Product
  Switch : Switch
  Switch1 : Switch  Criteria=u2 > Threshold
  Switch2 : Switch
  Switch3 : Switch  Criteria=u2 > Threshold
  Beta : Outport
  Temp : Outport  Port=2
  Alpha : Outport  Port=3
  wires:
  Q_out/1 -> Add/3
  Gain/1 -> Bias/1
  Divide1/1 -> Integrator/1  "dT/dt"
  Gain2/1 -> Product/1
  Integrator/1 -> Temp/1, Bias3/1, Bias2/1, Gain1/1  "T"
  Switch1/1 -> Divide1/1  "CON"
  Math Function1/1 -> Product/2
  Bias/1 -> Math Function1/1  "(1-Alpha)"
  Constant2/1 -> Switch2/3
  Add/1 -> Divide1/2  "CON*(dT/dt)"
  Gain5/1 -> Switch2/1, Switch2/2
  Switch2/1 -> Switch3/1, Bias4/1
  Constant/1 -> Switch/1
  Bias4/1 -> Gain6/1
  Switch/1 -> Switch1/1
  Switch3/1 -> Beta/1  "Beta"
  Gain6/1 -> Switch3/2
  Bias2/1 -> Gain5/1, Switch/2
  Constant4/1 -> Switch3/3
  Product/1 -> Add/1, Gain4/1  "-A*H_dr*exp()*(-Alhpa)"
  Gain1/1 -> Divide/1  "(-R*T)/Ea"
  Integrator1/1 -> Gain/1, Alpha/1  "Alpha"
  Gain4/1 -> Integrator1/1
  Constant3/1 -> Math Function1/2
  Constant1/1 -> Switch/3, Switch1/3
  Divide/1 -> Math Function/1  "Ea/(-R*T)"
  Math Function/1 -> Gain2/1
  Bias3/1 -> Gain3/1
  Gain3/1 -> Switch1/2
  Q_in/1 -> Add/2

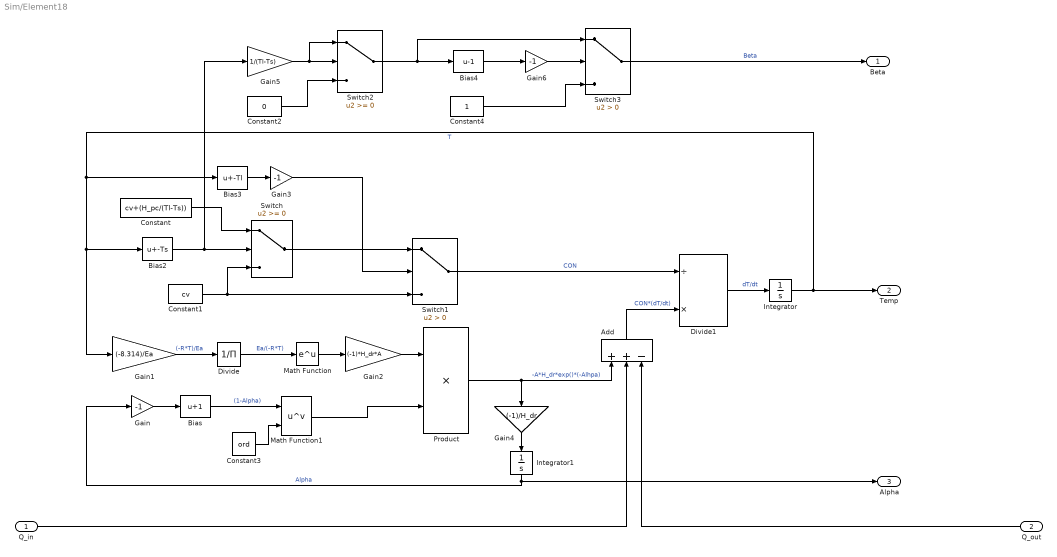
== system Sim/Element18 ==
  Q_in : Inport
  Q_out : Inport  Port=2
  Add : Sum  Inputs=++-
  Bias : Bias  Bias=1
  Bias2 : Bias  Bias=-Ts
  Bias3 : Bias  Bias=-Tl
  Bias4 : Bias  Bias=-1
  Constant : Constant  Value=cv+(H_pc/(Tl-Ts))
  Constant1 : Constant  Value=cv
  Constant2 : Constant  Value=0
  Constant3 : Constant  Value=ord
  Constant4 : Constant
  Divide : Product  Inputs=/
  Divide1 : Product  Inputs=/*
  Gain : Gain  Gain=-1
  Gain1 : Gain  Gain=(-8.314)/Ea
  Gain2 : Gain  Gain=(-1)*H_dr*A
  Gain3 : Gain  Gain=-1
  Gain4 : Gain  Gain=(-1)/H_dr
  Gain5 : Gain  Gain=1/(Tl-Ts)
  Gain6 : Gain  Gain=-1
  Integrator : Integrator  InitialCondition=T_0
  Integrator1 : Integrator
  Math Function : Math  SaturateOnIntegerOverflow=on
  Math Function1 : Math  Operator=pow  SaturateOnIntegerOverflow=on
  Product : Product
  Switch : Switch
  Switch1 : Switch  Criteria=u2 > Threshold
  Switch2 : Switch
  Switch3 : Switch  Criteria=u2 > Threshold
  Beta : Outport
  Temp : Outport  Port=2
  Alpha : Outport  Port=3
  wires:
  Q_out/1 -> Add/3
  Gain/1 -> Bias/1
  Divide1/1 -> Integrator/1  "dT/dt"
  Gain2/1 -> Product/1
  Integrator/1 -> Temp/1, Bias3/1, Bias2/1, Gain1/1  "T"
  Switch1/1 -> Divide1/1  "CON"
  Math Function1/1 -> Product/2
  Bias/1 -> Math Function1/1  "(1-Alpha)"
  Constant2/1 -> Switch2/3
  Add/1 -> Divide1/2  "CON*(dT/dt)"
  Gain5/1 -> Switch2/1, Switch2/2
  Switch2/1 -> Switch3/1, Bias4/1
  Constant/1 -> Switch/1
  Bias4/1 -> Gain6/1
  Switch/1 -> Switch1/1
  Switch3/1 -> Beta/1  "Beta"
  Gain6/1 -> Switch3/2
  Bias2/1 -> Gain5/1, Switch/2
  Constant4/1 -> Switch3/3
  Product/1 -> Add/1, Gain4/1  "-A*H_dr*exp()*(-Alhpa)"
  Gain1/1 -> Divide/1  "(-R*T)/Ea"
  Integrator1/1 -> Gain/1, Alpha/1  "Alpha"
  Gain4/1 -> Integrator1/1
  Constant3/1 -> Math Function1/2
  Constant1/1 -> Switch/3, Switch1/3
  Divide/1 -> Math Function/1  "Ea/(-R*T)"
  Math Function/1 -> Gain2/1
  Bias3/1 -> Gain3/1
  Gain3/1 -> Switch1/2
  Q_in/1 -> Add/2

== system Sim/Element19 ==
  Q_in : Inport
  Q_out : Inport  Port=2
  Add : Sum  Inputs=++-
  Bias : Bias  Bias=1
  Bias2 : Bias  Bias=-Ts
  Bias3 : Bias  Bias=-Tl
  Bias4 : Bias  Bias=-1
  Constant : Constant  Value=cv+(H_pc/(Tl-Ts))
  Constant1 : Constant  Value=cv
  Constant2 : Constant  Value=0
  Constant3 : Constant  Value=ord
  Constant4 : Constant
  Divide : Product  Inputs=/
  Divide1 : Product  Inputs=/*
  Gain : Gain  Gain=-1
  Gain1 : Gain  Gain=(-8.314)/Ea
  Gain2 : Gain  Gain=(-1)*H_dr*A
  Gain3 : Gain  Gain=-1
  Gain4 : Gain  Gain=(-1)/H_dr
  Gain5 : Gain  Gain=1/(Tl-Ts)
  Gain6 : Gain  Gain=-1
  Integrator : Integrator  InitialCondition=T_0
  Integrator1 : Integrator
  Math Function : Math  SaturateOnIntegerOverflow=on
  Math Function1 : Math  Operator=pow  SaturateOnIntegerOverflow=on
  Product : Product
  Switch : Switch
  Switch1 : Switch  Criteria=u2 > Threshold
  Switch2 : Switch
  Switch3 : Switch  Criteria=u2 > Threshold
  Beta : Outport
  Temp : Outport  Port=2
  Alpha : Outport  Port=3
  wires:
  Q_out/1 -> Add/3
  Gain/1 -> Bias/1
  Divide1/1 -> Integrator/1  "dT/dt"
  Gain2/1 -> Product/1
  Integrator/1 -> Temp/1, Bias3/1, Bias2/1, Gain1/1  "T"
  Switch1/1 -> Divide1/1  "CON"
  Math Function1/1 -> Product/2
  Bias/1 -> Math Function1/1  "(1-Alpha)"
  Constant2/1 -> Switch2/3
  Add/1 -> Divide1/2  "CON*(dT/dt)"
  Gain5/1 -> Switch2/1, Switch2/2
  Switch2/1 -> Switch3/1, Bias4/1
  Constant/1 -> Switch/1
  Bias4/1 -> Gain6/1
  Switch/1 -> Switch1/1
  Switch3/1 -> Beta/1  "Beta"
  Gain6/1 -> Switch3/2
  Bias2/1 -> Gain5/1, Switch/2
  Constant4/1 -> Switch3/3
  Product/1 -> Add/1, Gain4/1  "-A*H_dr*exp()*(-Alhpa)"
  Gain1/1 -> Divide/1  "(-R*T)/Ea"
  Integrator1/1 -> Gain/1, Alpha/1  "Alpha"
  Gain4/1 -> Integrator1/1
  Constant3/1 -> Math Function1/2
  Constant1/1 -> Switch/3, Switch1/3
  Divide/1 -> Math Function/1  "Ea/(-R*T)"
  Math Function/1 -> Gain2/1
  Bias3/1 -> Gain3/1
  Gain3/1 -> Switch1/2
  Q_in/1 -> Add/2

== system Sim/Element2 ==
  Q_in : Inport
  Q_out : Inport  Port=2
  Add : Sum  Inputs=++-
  Bias : Bias  Bias=1
  Bias2 : Bias  Bias=-Ts
  Bias3 : Bias  Bias=-Tl
  Bias4 : Bias  Bias=-1
  Constant : Constant  Value=cv+(H_pc/(Tl-Ts))
  Constant1 : Constant  Value=cv
  Constant2 : Constant  Value=0
  Constant3 : Constant  Value=ord
  Constant4 : Constant
  Divide : Product  Inputs=/
  Divide1 : Product  Inputs=/*
  Gain : Gain  Gain=-1
  Gain1 : Gain  Gain=(-8.314)/Ea
  Gain2 : Gain  Gain=(-1)*H_dr*A
  Gain3 : Gain  Gain=-1
  Gain4 : Gain  Gain=(-1)/H_dr
  Gain5 : Gain  Gain=1/(Tl-Ts)
  Gain6 : Gain  Gain=-1
  Integrator : Integrator  InitialCondition=T_0
  Integrator1 : Integrator
  Math Function : Math  SaturateOnIntegerOverflow=on
  Math Function1 : Math  Operator=pow  SaturateOnIntegerOverflow=on
  Product : Product
  Switch : Switch
  Switch1 : Switch  Criteria=u2 > Threshold
  Switch2 : Switch
  Switch3 : Switch  Criteria=u2 > Threshold
  Beta : Outport
  Temp : Outport  Port=2
  Alpha : Outport  Port=3
  wires:
  Q_out/1 -> Add/3
  Gain/1 -> Bias/1
  Divide1/1 -> Integrator/1  "dT/dt"
  Gain2/1 -> Product/1
  Integrator/1 -> Temp/1, Bias3/1, Bias2/1, Gain1/1  "T"
  Switch1/1 -> Divide1/1  "CON"
  Math Function1/1 -> Product/2
  Bias/1 -> Math Function1/1  "(1-Alpha)"
  Constant2/1 -> Switch2/3
  Add/1 -> Divide1/2  "CON*(dT/dt)"
  Gain5/1 -> Switch2/1, Switch2/2
  Switch2/1 -> Switch3/1, Bias4/1
  Constant/1 -> Switch/1
  Bias4/1 -> Gain6/1
  Switch/1 -> Switch1/1
  Switch3/1 -> Beta/1  "Beta"
  Gain6/1 -> Switch3/2
  Bias2/1 -> Gain5/1, Switch/2
  Constant4/1 -> Switch3/3
  Product/1 -> Add/1, Gain4/1  "-A*H_dr*exp()*(-Alhpa)"
  Gain1/1 -> Divide/1  "(-R*T)/Ea"
  Integrator1/1 -> Gain/1, Alpha/1  "Alpha"
  Gain4/1 -> Integrator1/1
  Constant3/1 -> Math Function1/2
  Constant1/1 -> Switch/3, Switch1/3
  Divide/1 -> Math Function/1  "Ea/(-R*T)"
  Math Function/1 -> Gain2/1
  Bias3/1 -> Gain3/1
  Gain3/1 -> Switch1/2
  Q_in/1 -> Add/2

== system Sim/Element20 ==
  Q_in : Inport
  Q_out : Inport  Port=2
  Add : Sum  Inputs=++-
  Bias : Bias  Bias=1
  Bias2 : Bias  Bias=-Ts
  Bias3 : Bias  Bias=-Tl
  Bias4 : Bias  Bias=-1
  Constant : Constant  Value=cv+(H_pc/(Tl-Ts))
  Constant1 : Constant  Value=cv
  Constant2 : Constant  Value=0
  Constant3 : Constant  Value=ord
  Constant4 : Constant
  Divide : Product  Inputs=/
  Divide1 : Product  Inputs=/*
  Gain : Gain  Gain=-1
  Gain1 : Gain  Gain=(-8.314)/Ea
  Gain2 : Gain  Gain=(-1)*H_dr*A
  Gain3 : Gain  Gain=-1
  Gain4 : Gain  Gain=(-1)/H_dr
  Gain5 : Gain  Gain=1/(Tl-Ts)
  Gain6 : Gain  Gain=-1
  Integrator : Integrator  InitialCondition=T_0
  Integrator1 : Integrator
  Math Function : Math  SaturateOnIntegerOverflow=on
  Math Function1 : Math  Operator=pow  SaturateOnIntegerOverflow=on
  Product : Product
  Switch : Switch
  Switch1 : Switch  Criteria=u2 > Threshold
  Switch2 : Switch
  Switch3 : Switch  Criteria=u2 > Threshold
  Beta : Outport
  Temp : Outport  Port=2
  Alpha : Outport  Port=3
  wires:
  Q_out/1 -> Add/3
  Gain/1 -> Bias/1
  Divide1/1 -> Integrator/1  "dT/dt"
  Gain2/1 -> Product/1
  Integrator/1 -> Temp/1, Bias3/1, Bias2/1, Gain1/1  "T"
  Switch1/1 -> Divide1/1  "CON"
  Math Function1/1 -> Product/2
  Bias/1 -> Math Function1/1  "(1-Alpha)"
  Constant2/1 -> Switch2/3
  Add/1 -> Divide1/2  "CON*(dT/dt)"
  Gain5/1 -> Switch2/1, Switch2/2
  Switch2/1 -> Switch3/1, Bias4/1
  Constant/1 -> Switch/1
  Bias4/1 -> Gain6/1
  Switch/1 -> Switch1/1
  Switch3/1 -> Beta/1  "Beta"
  Gain6/1 -> Switch3/2
  Bias2/1 -> Gain5/1, Switch/2
  Constant4/1 -> Switch3/3
  Product/1 -> Add/1, Gain4/1  "-A*H_dr*exp()*(-Alhpa)"
  Gain1/1 -> Divide/1  "(-R*T)/Ea"
  Integrator1/1 -> Gain/1, Alpha/1  "Alpha"
  Gain4/1 -> Integrator1/1
  Constant3/1 -> Math Function1/2
  Constant1/1 -> Switch/3, Switch1/3
  Divide/1 -> Math Function/1  "Ea/(-R*T)"
  Math Function/1 -> Gain2/1
  Bias3/1 -> Gain3/1
  Gain3/1 -> Switch1/2
  Q_in/1 -> Add/2

== system Sim/Element21 ==
  Q_in : Inport
  Q_out : Inport  Port=2
  Add : Sum  Inputs=++-
  Bias : Bias  Bias=1
  Bias2 : Bias  Bias=-Ts
  Bias3 : Bias  Bias=-Tl
  Bias4 : Bias  Bias=-1
  Constant : Constant  Value=cv+(H_pc/(Tl-Ts))
  Constant1 : Constant  Value=cv
  Constant2 : Constant  Value=0
  Constant3 : Constant  Value=ord
  Constant4 : Constant
  Divide : Product  Inputs=/
  Divide1 : Product  Inputs=/*
  Gain : Gain  Gain=-1
  Gain1 : Gain  Gain=(-8.314)/Ea
  Gain2 : Gain  Gain=(-1)*H_dr*A
  Gain3 : Gain  Gain=-1
  Gain4 : Gain  Gain=(-1)/H_dr
  Gain5 : Gain  Gain=1/(Tl-Ts)
  Gain6 : Gain  Gain=-1
  Integrator : Integrator  InitialCondition=T_0
  Integrator1 : Integrator
  Math Function : Math  SaturateOnIntegerOverflow=on
  Math Function1 : Math  Operator=pow  SaturateOnIntegerOverflow=on
  Product : Product
  Switch : Switch
  Switch1 : Switch  Criteria=u2 > Threshold
  Switch2 : Switch
  Switch3 : Switch  Criteria=u2 > Threshold
  Beta : Outport
  Temp : Outport  Port=2
  Alpha : Outport  Port=3
  wires:
  Q_out/1 -> Add/3
  Gain/1 -> Bias/1
  Divide1/1 -> Integrator/1  "dT/dt"
  Gain2/1 -> Product/1
  Integrator/1 -> Temp/1, Bias3/1, Bias2/1, Gain1/1  "T"
  Switch1/1 -> Divide1/1  "CON"
  Math Function1/1 -> Product/2
  Bias/1 -> Math Function1/1  "(1-Alpha)"
  Constant2/1 -> Switch2/3
  Add/1 -> Divide1/2  "CON*(dT/dt)"
  Gain5/1 -> Switch2/1, Switch2/2
  Switch2/1 -> Switch3/1, Bias4/1
  Constant/1 -> Switch/1
  Bias4/1 -> Gain6/1
  Switch/1 -> Switch1/1
  Switch3/1 -> Beta/1  "Beta"
  Gain6/1 -> Switch3/2
  Bias2/1 -> Gain5/1, Switch/2
  Constant4/1 -> Switch3/3
  Product/1 -> Add/1, Gain4/1  "-A*H_dr*exp()*(-Alhpa)"
  Gain1/1 -> Divide/1  "(-R*T)/Ea"
  Integrator1/1 -> Gain/1, Alpha/1  "Alpha"
  Gain4/1 -> Integrator1/1
  Constant3/1 -> Math Function1/2
  Constant1/1 -> Switch/3, Switch1/3
  Divide/1 -> Math Function/1  "Ea/(-R*T)"
  Math Function/1 -> Gain2/1
  Bias3/1 -> Gain3/1
  Gain3/1 -> Switch1/2
  Q_in/1 -> Add/2

== system Sim/Element22 ==
  Q_in : Inport
  Q_out : Inport  Port=2
  Add : Sum  Inputs=++-
  Bias : Bias  Bias=1
  Bias2 : Bias  Bias=-Ts
  Bias3 : Bias  Bias=-Tl
  Bias4 : Bias  Bias=-1
  Constant : Constant  Value=cv+(H_pc/(Tl-Ts))
  Constant1 : Constant  Value=cv
  Constant2 : Constant  Value=0
  Constant3 : Constant  Value=ord
  Constant4 : Constant
  Divide : Product  Inputs=/
  Divide1 : Product  Inputs=/*
  Gain : Gain  Gain=-1
  Gain1 : Gain  Gain=(-8.314)/Ea
  Gain2 : Gain  Gain=(-1)*H_dr*A
  Gain3 : Gain  Gain=-1
  Gain4 : Gain  Gain=(-1)/H_dr
  Gain5 : Gain  Gain=1/(Tl-Ts)
  Gain6 : Gain  Gain=-1
  Integrator : Integrator  InitialCondition=T_0
  Integrator1 : Integrator
  Math Function : Math  SaturateOnIntegerOverflow=on
  Math Function1 : Math  Operator=pow  SaturateOnIntegerOverflow=on
  Product : Product
  Switch : Switch
  Switch1 : Switch  Criteria=u2 > Threshold
  Switch2 : Switch
  Switch3 : Switch  Criteria=u2 > Threshold
  Beta : Outport
  Temp : Outport  Port=2
  Alpha : Outport  Port=3
  wires:
  Q_out/1 -> Add/3
  Gain/1 -> Bias/1
  Divide1/1 -> Integrator/1  "dT/dt"
  Gain2/1 -> Product/1
  Integrator/1 -> Temp/1, Bias3/1, Bias2/1, Gain1/1  "T"
  Switch1/1 -> Divide1/1  "CON"
  Math Function1/1 -> Product/2
  Bias/1 -> Math Function1/1  "(1-Alpha)"
  Constant2/1 -> Switch2/3
  Add/1 -> Divide1/2  "CON*(dT/dt)"
  Gain5/1 -> Switch2/1, Switch2/2
  Switch2/1 -> Switch3/1, Bias4/1
  Constant/1 -> Switch/1
  Bias4/1 -> Gain6/1
  Switch/1 -> Switch1/1
  Switch3/1 -> Beta/1  "Beta"
  Gain6/1 -> Switch3/2
  Bias2/1 -> Gain5/1, Switch/2
  Constant4/1 -> Switch3/3
  Product/1 -> Add/1, Gain4/1  "-A*H_dr*exp()*(-Alhpa)"
  Gain1/1 -> Divide/1  "(-R*T)/Ea"
  Integrator1/1 -> Gain/1, Alpha/1  "Alpha"
  Gain4/1 -> Integrator1/1
  Constant3/1 -> Math Function1/2
  Constant1/1 -> Switch/3, Switch1/3
  Divide/1 -> Math Function/1  "Ea/(-R*T)"
  Math Function/1 -> Gain2/1
  Bias3/1 -> Gain3/1
  Gain3/1 -> Switch1/2
  Q_in/1 -> Add/2

== system Sim/Element23 ==
  Q_in : Inport
  Q_out : Inport  Port=2
  Add : Sum  Inputs=++-
  Bias : Bias  Bias=1
  Bias2 : Bias  Bias=-Ts
  Bias3 : Bias  Bias=-Tl
  Bias4 : Bias  Bias=-1
  Constant : Constant  Value=cv+(H_pc/(Tl-Ts))
  Constant1 : Constant  Value=cv
  Constant2 : Constant  Value=0
  Constant3 : Constant  Value=ord
  Constant4 : Constant
  Divide : Product  Inputs=/
  Divide1 : Product  Inputs=/*
  Gain : Gain  Gain=-1
  Gain1 : Gain  Gain=(-8.314)/Ea
  Gain2 : Gain  Gain=(-1)*H_dr*A
  Gain3 : Gain  Gain=-1
  Gain4 : Gain  Gain=(-1)/H_dr
  Gain5 : Gain  Gain=1/(Tl-Ts)
  Gain6 : Gain  Gain=-1
  Integrator : Integrator  InitialCondition=T_0
  Integrator1 : Integrator
  Math Function : Math  SaturateOnIntegerOverflow=on
  Math Function1 : Math  Operator=pow  SaturateOnIntegerOverflow=on
  Product : Product
  Switch : Switch
  Switch1 : Switch  Criteria=u2 > Threshold
  Switch2 : Switch
  Switch3 : Switch  Criteria=u2 > Threshold
  Beta : Outport
  Temp : Outport  Port=2
  Alpha : Outport  Port=3
  wires:
  Q_out/1 -> Add/3
  Gain/1 -> Bias/1
  Divide1/1 -> Integrator/1  "dT/dt"
  Gain2/1 -> Product/1
  Integrator/1 -> Temp/1, Bias3/1, Bias2/1, Gain1/1  "T"
  Switch1/1 -> Divide1/1  "CON"
  Math Function1/1 -> Product/2
  Bias/1 -> Math Function1/1  "(1-Alpha)"
  Constant2/1 -> Switch2/3
  Add/1 -> Divide1/2  "CON*(dT/dt)"
  Gain5/1 -> Switch2/1, Switch2/2
  Switch2/1 -> Switch3/1, Bias4/1
  Constant/1 -> Switch/1
  Bias4/1 -> Gain6/1
  Switch/1 -> Switch1/1
  Switch3/1 -> Beta/1  "Beta"
  Gain6/1 -> Switch3/2
  Bias2/1 -> Gain5/1, Switch/2
  Constant4/1 -> Switch3/3
  Product/1 -> Add/1, Gain4/1  "-A*H_dr*exp()*(-Alhpa)"
  Gain1/1 -> Divide/1  "(-R*T)/Ea"
  Integrator1/1 -> Gain/1, Alpha/1  "Alpha"
  Gain4/1 -> Integrator1/1
  Constant3/1 -> Math Function1/2
  Constant1/1 -> Switch/3, Switch1/3
  Divide/1 -> Math Function/1  "Ea/(-R*T)"
  Math Function/1 -> Gain2/1
  Bias3/1 -> Gain3/1
  Gain3/1 -> Switch1/2
  Q_in/1 -> Add/2

== system Sim/Element24 ==
  Q_in : Inport
  Q_out : Inport  Port=2
  Add : Sum  Inputs=++-
  Bias : Bias  Bias=1
  Bias2 : Bias  Bias=-Ts
  Bias3 : Bias  Bias=-Tl
  Bias4 : Bias  Bias=-1
  Constant : Constant  Value=cv+(H_pc/(Tl-Ts))
  Constant1 : Constant  Value=cv
  Constant2 : Constant  Value=0
  Constant3 : Constant  Value=ord
  Constant4 : Constant
  Divide : Product  Inputs=/
  Divide1 : Product  Inputs=/*
  Gain : Gain  Gain=-1
  Gain1 : Gain  Gain=(-8.314)/Ea
  Gain2 : Gain  Gain=(-1)*H_dr*A
  Gain3 : Gain  Gain=-1
  Gain4 : Gain  Gain=(-1)/H_dr
  Gain5 : Gain  Gain=1/(Tl-Ts)
  Gain6 : Gain  Gain=-1
  Integrator : Integrator  InitialCondition=T_0
  Integrator1 : Integrator
  Math Function : Math  SaturateOnIntegerOverflow=on
  Math Function1 : Math  Operator=pow  SaturateOnIntegerOverflow=on
  Product : Product
  Switch : Switch
  Switch1 : Switch  Criteria=u2 > Threshold
  Switch2 : Switch
  Switch3 : Switch  Criteria=u2 > Threshold
  Beta : Outport
  Temp : Outport  Port=2
  Alpha : Outport  Port=3
  wires:
  Q_out/1 -> Add/3
  Gain/1 -> Bias/1
  Divide1/1 -> Integrator/1  "dT/dt"
  Gain2/1 -> Product/1
  Integrator/1 -> Temp/1, Bias3/1, Bias2/1, Gain1/1  "T"
  Switch1/1 -> Divide1/1  "CON"
  Math Function1/1 -> Product/2
  Bias/1 -> Math Function1/1  "(1-Alpha)"
  Constant2/1 -> Switch2/3
  Add/1 -> Divide1/2  "CON*(dT/dt)"
  Gain5/1 -> Switch2/1, Switch2/2
  Switch2/1 -> Switch3/1, Bias4/1
  Constant/1 -> Switch/1
  Bias4/1 -> Gain6/1
  Switch/1 -> Switch1/1
  Switch3/1 -> Beta/1  "Beta"
  Gain6/1 -> Switch3/2
  Bias2/1 -> Gain5/1, Switch/2
  Constant4/1 -> Switch3/3
  Product/1 -> Add/1, Gain4/1  "-A*H_dr*exp()*(-Alhpa)"
  Gain1/1 -> Divide/1  "(-R*T)/Ea"
  Integrator1/1 -> Gain/1, Alpha/1  "Alpha"
  Gain4/1 -> Integrator1/1
  Constant3/1 -> Math Function1/2
  Constant1/1 -> Switch/3, Switch1/3
  Divide/1 -> Math Function/1  "Ea/(-R*T)"
  Math Function/1 -> Gain2/1
  Bias3/1 -> Gain3/1
  Gain3/1 -> Switch1/2
  Q_in/1 -> Add/2

== system Sim/Element25 ==
  Q_in : Inport
  Q_out : Inport  Port=2
  Add : Sum  Inputs=++-
  Bias : Bias  Bias=1
  Bias2 : Bias  Bias=-Ts
  Bias3 : Bias  Bias=-Tl
  Bias4 : Bias  Bias=-1
  Constant : Constant  Value=cv+(H_pc/(Tl-Ts))
  Constant1 : Constant  Value=cv
  Constant2 : Constant  Value=0
  Constant3 : Constant  Value=ord
  Constant4 : Constant
  Divide : Product  Inputs=/
  Divide1 : Product  Inputs=/*
  Gain : Gain  Gain=-1
  Gain1 : Gain  Gain=(-8.314)/Ea
  Gain2 : Gain  Gain=(-1)*H_dr*A
  Gain3 : Gain  Gain=-1
  Gain4 : Gain  Gain=(-1)/H_dr
  Gain5 : Gain  Gain=1/(Tl-Ts)
  Gain6 : Gain  Gain=-1
  Integrator : Integrator  InitialCondition=T_0
  Integrator1 : Integrator
  Math Function : Math  SaturateOnIntegerOverflow=on
  Math Function1 : Math  Operator=pow  SaturateOnIntegerOverflow=on
  Product : Product
  Switch : Switch
  Switch1 : Switch  Criteria=u2 > Threshold
  Switch2 : Switch
  Switch3 : Switch  Criteria=u2 > Threshold
  Beta : Outport
  Temp : Outport  Port=2
  Alpha : Outport  Port=3
  wires:
  Q_out/1 -> Add/3
  Gain/1 -> Bias/1
  Divide1/1 -> Integrator/1  "dT/dt"
  Gain2/1 -> Product/1
  Integrator/1 -> Temp/1, Bias3/1, Bias2/1, Gain1/1  "T"
  Switch1/1 -> Divide1/1  "CON"
  Math Function1/1 -> Product/2
  Bias/1 -> Math Function1/1  "(1-Alpha)"
  Constant2/1 -> Switch2/3
  Add/1 -> Divide1/2  "CON*(dT/dt)"
  Gain5/1 -> Switch2/1, Switch2/2
  Switch2/1 -> Switch3/1, Bias4/1
  Constant/1 -> Switch/1
  Bias4/1 -> Gain6/1
  Switch/1 -> Switch1/1
  Switch3/1 -> Beta/1  "Beta"
  Gain6/1 -> Switch3/2
  Bias2/1 -> Gain5/1, Switch/2
  Constant4/1 -> Switch3/3
  Product/1 -> Add/1, Gain4/1  "-A*H_dr*exp()*(-Alhpa)"
  Gain1/1 -> Divide/1  "(-R*T)/Ea"
  Integrator1/1 -> Gain/1, Alpha/1  "Alpha"
  Gain4/1 -> Integrator1/1
  Constant3/1 -> Math Function1/2
  Constant1/1 -> Switch/3, Switch1/3
  Divide/1 -> Math Function/1  "Ea/(-R*T)"
  Math Function/1 -> Gain2/1
  Bias3/1 -> Gain3/1
  Gain3/1 -> Switch1/2
  Q_in/1 -> Add/2

== system Sim/Element26 ==
  Q_in : Inport
  Q_out : Inport  Port=2
  Add : Sum  Inputs=++-
  Bias : Bias  Bias=1
  Bias2 : Bias  Bias=-Ts
  Bias3 : Bias  Bias=-Tl
  Bias4 : Bias  Bias=-1
  Constant : Constant  Value=cv+(H_pc/(Tl-Ts))
  Constant1 : Constant  Value=cv
  Constant2 : Constant  Value=0
  Constant3 : Constant  Value=ord
  Constant4 : Constant
  Divide : Product  Inputs=/
  Divide1 : Product  Inputs=/*
  Gain : Gain  Gain=-1
  Gain1 : Gain  Gain=(-8.314)/Ea
  Gain2 : Gain  Gain=(-1)*H_dr*A
  Gain3 : Gain  Gain=-1
  Gain4 : Gain  Gain=(-1)/H_dr
  Gain5 : Gain  Gain=1/(Tl-Ts)
  Gain6 : Gain  Gain=-1
  Integrator : Integrator  InitialCondition=T_0
  Integrator1 : Integrator
  Math Function : Math  SaturateOnIntegerOverflow=on
  Math Function1 : Math  Operator=pow  SaturateOnIntegerOverflow=on
  Product : Product
  Switch : Switch
  Switch1 : Switch  Criteria=u2 > Threshold
  Switch2 : Switch
  Switch3 : Switch  Criteria=u2 > Threshold
  Beta : Outport
  Temp : Outport  Port=2
  Alpha : Outport  Port=3
  wires:
  Q_out/1 -> Add/3
  Gain/1 -> Bias/1
  Divide1/1 -> Integrator/1  "dT/dt"
  Gain2/1 -> Product/1
  Integrator/1 -> Temp/1, Bias3/1, Bias2/1, Gain1/1  "T"
  Switch1/1 -> Divide1/1  "CON"
  Math Function1/1 -> Product/2
  Bias/1 -> Math Function1/1  "(1-Alpha)"
  Constant2/1 -> Switch2/3
  Add/1 -> Divide1/2  "CON*(dT/dt)"
  Gain5/1 -> Switch2/1, Switch2/2
  Switch2/1 -> Switch3/1, Bias4/1
  Constant/1 -> Switch/1
  Bias4/1 -> Gain6/1
  Switch/1 -> Switch1/1
  Switch3/1 -> Beta/1  "Beta"
  Gain6/1 -> Switch3/2
  Bias2/1 -> Gain5/1, Switch/2
  Constant4/1 -> Switch3/3
  Product/1 -> Add/1, Gain4/1  "-A*H_dr*exp()*(-Alhpa)"
  Gain1/1 -> Divide/1  "(-R*T)/Ea"
  Integrator1/1 -> Gain/1, Alpha/1  "Alpha"
  Gain4/1 -> Integrator1/1
  Constant3/1 -> Math Function1/2
  Constant1/1 -> Switch/3, Switch1/3
  Divide/1 -> Math Function/1  "Ea/(-R*T)"
  Math Function/1 -> Gain2/1
  Bias3/1 -> Gain3/1
  Gain3/1 -> Switch1/2
  Q_in/1 -> Add/2
